simulink model "sampleModel1714_4"  (R2023a)
settings: Solver=VariableStepAuto  StartTime=0.0  StopTime=10.0  RelTol=1e-3
libraries: hdlsllib x5, simulink x2
settings Model: Creator=user1  LastModifiedBy=user1

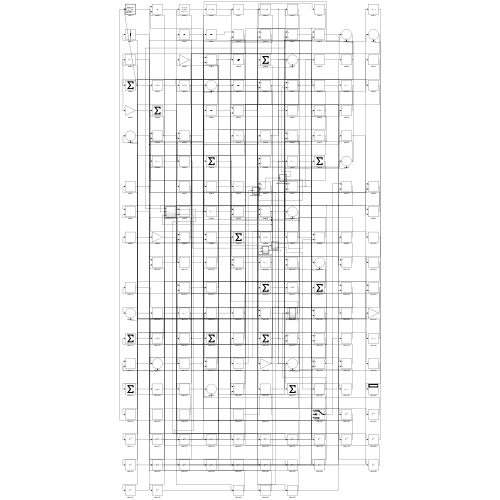
[thumbnail: Simulink's stored preview of the top-level diagram]
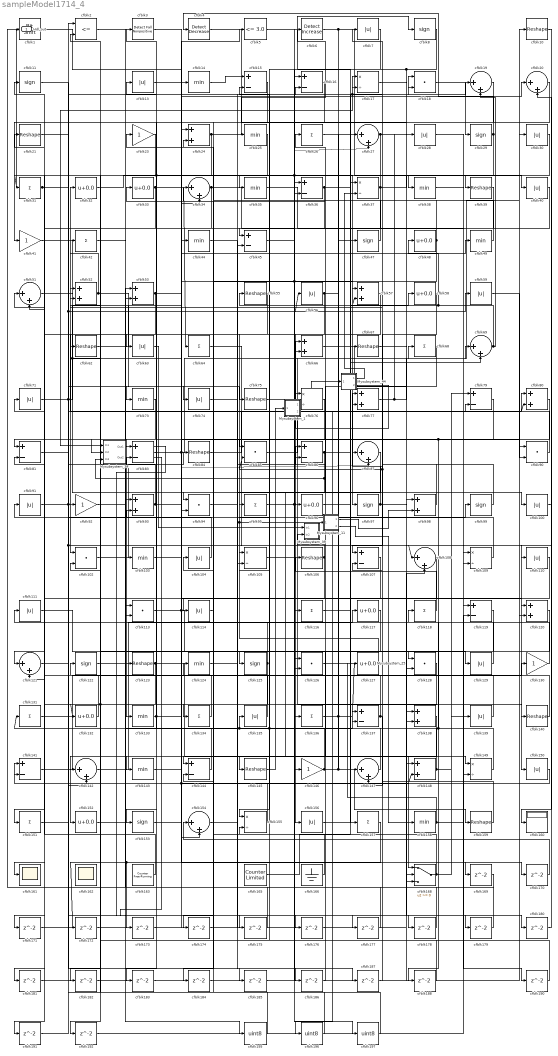
== system sampleModel1714_4 ==
  Mysubsystem_1 : Subsystem  TreatAsAtomicUnit=on  RTWFcnName=Mysubsystem_1
      settings: RTWFcnNameOpts=User specified  RTWFileNameOpts=Use function name
  Mysubsystem_11 : Subsystem  TreatAsAtomicUnit=on  RTWFcnName=Mysubsystem_11
      settings: RTWFcnNameOpts=User specified  RTWFileNameOpts=Use function name
  Mysubsystem_25 : Subsystem  TreatAsAtomicUnit=on  RTWFcnName=Mysubsystem_25
      settings: RTWFcnNameOpts=User specified  RTWFileNameOpts=Use function name
  Mysubsystem_34 : Subsystem  TreatAsAtomicUnit=on  RTWFcnName=Mysubsystem_34
      settings: RTWFcnNameOpts=User specified  RTWFileNameOpts=Use function name
  Mysubsystem_39 : Subsystem  TreatAsAtomicUnit=on  RTWFcnName=Mysubsystem_39
      settings: RTWFcnNameOpts=User specified  RTWFileNameOpts=Use function name
  Mysubsystem_44 : Subsystem  TreatAsAtomicUnit=on  RTWFcnName=Mysubsystem_44
      settings: RTWFcnNameOpts=User specified  RTWFileNameOpts=Use function name
  cfblk1 : hdlsllib/Logic and Bit Operations/Bit Shift  mode=Shift Left Logical  N=0
  cfblk{10,21,39,55,62,67,75,84,106,123,140,145,159} (13 alike) : Reshape
  cfblk{7,13,28,30,40,56,59,63,71,74,91,100,104,110..111,114,129,135,139,150,156} (21 alike) : Abs  OutDataTypeStr=uint8  SaturateOnIntegerOverflow=off
  cfblk{18,85,90,94,102,113,126,128} (8 alike) : DotProduct  OutDataTypeStr=uint8
  cfblk{14,25,35,38,44,49,73,103,124,133,143,158} (12 alike) : MinMax  OutDataTypeStr=uint8
  cfblk{17,37,76,105,109,149,155} (7 alike) : Product  Inputs=*/  OutDataTypeStr=uint8  RndMeth=Zero  SaturateOnIntegerOverflow=on
  cfblk{15..16,36,45,79,81,83,86,107,119,137,141,144} (13 alike) : Sum  Inputs=+-  OutDataTypeStr=uint8
  cfblk{19..20,27,34,51,69,87,108,121,142,147,154} (12 alike) : Sum  Inputs=|++  OutDataTypeStr=uint8
  cfblk{8,11,29,47,97,99,122,125,153} (9 alike) : Signum
  cfblk{26,31,42,64,68,95,116,118,131,134,136,151,157} (13 alike) : Sum  Inputs=+  OutDataTypeStr=uint8
  cfblk{32..33,48,58,96,117,127,132,152} (9 alike) : Bias  Bias=0.0  SaturateOnIntegerOverflow=off
  cfblk{24,52..53,57,66,77,80,93,98,120,138,148} (12 alike) : Sum  OutDataTypeStr=uint8
  cfblk{23,41,92,130,146} (5 alike) : Gain  OutDataTypeStr=uint8
  cfblk160 : Display
  cfblk161 : Scope
  cfblk162 : Scope
      settings: Floating=on
  cfblk163 : hdlsllib/Sources/Counter Free-Running  NumBits=16  tsamp=-1
  cfblk165 : hdlsllib/Sources/Counter Limited  uplimit=7  tsamp=-1
  cfblk166 : Ground
  cfblk168 : Switch  OutDataTypeStr=uint8  SaturateOnIntegerOverflow=off  InputSameDT=off
  cfblk{169..188,190..192} (23 alike) : Delay  SampleTime=1
  cfblk195 : DataTypeConversion  OutDataTypeStr=uint8  SaturateOnIntegerOverflow=off  RndMeth=Floor
  cfblk196 : DataTypeConversion  OutDataTypeStr=uint8  SaturateOnIntegerOverflow=off  RndMeth=Floor
  cfblk197 : DataTypeConversion  OutDataTypeStr=uint8  SaturateOnIntegerOverflow=off  RndMeth=Floor
  cfblk2 : RelationalOperator  Operator=<=  OutDataTypeStr=boolean  InputSameDT=off
  cfblk3 : hdlsllib/Logic and Bit Operations/Detect Fall Nonpositive  vinit=0  OutDataTypeStr=uint8
  cfblk4 : simulink/Logic and Bit Operations/Detect Decrease  vinit=0.0  OutDataTypeStr=uint8
      settings: LibrarySourceBlock=|
      | hdlsllib/Logic and Bit
      | Operations/Detect
      | Decrease
  cfblk5 : hdlsllib/Logic and Bit Operations/Compare To Constant  relop=<=  const=3.0  OutDataTypeStr=uint8
  cfblk6 : simulink/Logic and Bit Operations/Detect Increase  vinit=0.0  OutDataTypeStr=uint8
      settings: LibrarySourceBlock=|
      | hdlsllib/Logic and Bit
      | Operations/Detect
      | Increase
  Hdl_out : Outport  OutDataTypeStr=uint8
  wires:
  cfblk86/1 -> Mysubsystem_34/3(In3), cfblk144/1, cfblk18/2
  cfblk6/1 -> cfblk38/1, cfblk147/1
  cfblk53/1 -> cfblk102/1, cfblk90/2
  cfblk109/1 -> cfblk33/1
  cfblk32/1 -> cfblk97/1
  cfblk150/1 -> cfblk141/1
  cfblk33/1 -> cfblk64/1, cfblk51/2
  cfblk31/1 -> cfblk108/1, cfblk176/1, Hdl_out/1
  cfblk48/1 -> cfblk76/2, cfblk174/1, cfblk24/2
  cfblk142/1 -> cfblk117/1
  cfblk151/1 -> cfblk56/1, cfblk17/2, cfblk92/1
  cfblk114/1 -> cfblk34/1
  cfblk165/1 -> cfblk37/1
  cfblk41/1 -> cfblk73/1
  cfblk137/1 -> cfblk122/1, cfblk147/2
  cfblk129/1 -> cfblk71/1
  cfblk84/1 -> cfblk77/1
  cfblk100/1 -> cfblk160/1
  cfblk121/1 -> cfblk99/1
  cfblk123/1 -> cfblk168/1, cfblk191/1
  cfblk163/1 -> cfblk51/1
  cfblk166/1 -> cfblk105/1
  cfblk57/1 -> cfblk156/1
  cfblk96/1 -> cfblk58/1
  cfblk64/1 -> cfblk150/1
  cfblk87/1 -> cfblk105/2
  cfblk136/1 -> cfblk127/1, cfblk47/1
  cfblk25/1 -> cfblk143/1, cfblk161/1
  cfblk158/1 -> Mysubsystem_25/1(In1), cfblk130/1
  cfblk133/1 -> cfblk13/1, cfblk5/1
  cfblk24/1 -> cfblk8/1, cfblk63/1
  cfblk83/1 -> cfblk25/1, cfblk59/1
  cfblk29/1 -> cfblk4/1, cfblk182/1
  cfblk58/1 -> cfblk107/1
  cfblk26/1 -> cfblk39/1
  cfblk90/1 -> cfblk32/1
  cfblk135/1 -> cfblk91/1
  cfblk138/1 -> cfblk152/1
  cfblk75/1 -> cfblk140/1
  cfblk19/1 -> cfblk41/1
  cfblk10/1 -> cfblk110/1
  cfblk140/1 -> cfblk111/1
  cfblk159/1 -> cfblk52/1, cfblk85/2
  cfblk102/1 -> cfblk84/1
  cfblk108/1 -> cfblk125/1
  cfblk73/1 -> cfblk133/1
  cfblk113/1 -> cfblk128/1, cfblk87/2
  cfblk149/1 -> cfblk131/1, cfblk135/1, cfblk118/1
  cfblk59/1 -> cfblk90/1
  cfblk55/1 -> cfblk114/1
  cfblk42/1 -> cfblk103/1
  cfblk93/1 -> cfblk62/1, cfblk169/1
  cfblk141/1 -> cfblk30/1
  cfblk99/1 -> cfblk55/1
  cfblk85/1 -> cfblk10/1
  cfblk18/1 -> cfblk29/1
  cfblk39/1 -> cfblk155/1
  cfblk51/1 -> cfblk94/1
  cfblk111/1 -> cfblk126/1
  cfblk71/1 -> cfblk14/1, cfblk44/1, cfblk79/2
  cfblk118/1 -> cfblk106/1
  cfblk168/1 -> cfblk124/1, cfblk79/1
  cfblk21/1 -> cfblk75/1
  cfblk74/1 -> cfblk68/1
  cfblk4/1 -> cfblk98/1
  cfblk126/1 -> cfblk80/1
  cfblk52/1 -> cfblk74/1, cfblk42/1
  cfblk23/1 -> cfblk53/2
  cfblk56/1 -> cfblk81/1, cfblk27/1
  cfblk5/1 -> cfblk157/1
  cfblk148/1 -> cfblk95/1, cfblk121/2, cfblk139/1
  cfblk38/1 -> cfblk119/1
  cfblk45/1 -> cfblk6/1
  cfblk127/1 -> cfblk107/2
  cfblk77/1 -> cfblk69/1, cfblk28/1
  cfblk97/1 -> cfblk77/2, cfblk109/2
  cfblk105/1 -> cfblk19/1, cfblk80/2
  cfblk153/1 -> cfblk49/1, cfblk148/2
  cfblk154/1 -> cfblk16/2
  cfblk124/1 -> cfblk86/1
  cfblk30/1 -> cfblk31/1, cfblk36/2
  cfblk69/1 -> cfblk48/1, cfblk57/2, cfblk19/2
  cfblk139/1 -> cfblk87/1
  cfblk62/1 -> cfblk20/1
  cfblk103/1 -> cfblk120/1
  cfblk47/1 -> cfblk23/1
  cfblk146/1 -> cfblk67/1, cfblk159/1, cfblk93/2
  cfblk144/1 -> cfblk52/2
  cfblk134/1 -> cfblk81/2
  cfblk27/1 -> cfblk180/1, cfblk181/1
  cfblk132/1 -> cfblk21/1
  cfblk17/1 -> cfblk148/1
  cfblk36/1 -> cfblk85/1, cfblk129/1
  cfblk143/1 -> cfblk76/1
  cfblk98/1 -> Mysubsystem_34/1(In1), cfblk17/1
  cfblk125/1 -> cfblk3/1, cfblk183/1
  cfblk1/1 -> cfblk154/2
  cfblk131/1 -> cfblk116/1
  cfblk104/1 -> cfblk11/1
  cfblk15/1 -> cfblk134/1
  cfblk147/1 -> cfblk26/1
  cfblk40/1 -> cfblk83/1
  cfblk156/1 -> cfblk18/1
  cfblk67/1 -> cfblk149/1
  cfblk20/1 -> cfblk123/1
  cfblk95/1 -> cfblk27/2, cfblk197/1
  cfblk3/1 -> cfblk57/1
  cfblk106/1 -> Mysubsystem_39/2(In2), cfblk192/1
  cfblk7/1 -> cfblk45/1
  cfblk155/1 -> cfblk141/2
  cfblk68/1 -> cfblk96/1
  cfblk79/1 -> cfblk151/1, cfblk188/1
  cfblk107/1 -> cfblk121/1
  cfblk80/1 -> cfblk94/2
  cfblk116/1 -> cfblk69/2
  cfblk14/1 -> cfblk15/1
  cfblk49/1 -> cfblk7/1
  cfblk16/1 -> cfblk153/1
  cfblk37/1 -> cfblk40/1, cfblk35/1, cfblk145/1
  cfblk130/1 -> cfblk15/2
  cfblk120/1 -> cfblk136/1
  cfblk13/1 -> cfblk100/1
  cfblk152/1 -> cfblk137/1
  cfblk66/1 -> cfblk138/2
  cfblk119/1 -> cfblk142/1, cfblk132/1
  cfblk157/1 -> cfblk172/1, cfblk173/1
  cfblk35/1 -> cfblk109/1
  cfblk8/1 -> cfblk128/2, cfblk66/2
  cfblk91/1 -> cfblk83/2
  cfblk117/1 -> cfblk146/1
  cfblk34/1 -> cfblk126/2, cfblk113/2
  cfblk169/1 -> cfblk1/1
  cfblk94/1 -> cfblk170/1
  cfblk170/1 -> cfblk154/1
  cfblk128/1 -> cfblk171/1
  cfblk171/1 -> cfblk34/2
  cfblk172/1 -> cfblk45/2
  cfblk173/1 -> cfblk168/2
  cfblk174/1 -> cfblk144/2
  cfblk122/1 -> cfblk175/1
  cfblk175/1 -> cfblk24/1
  cfblk176/1 -> cfblk138/1
  cfblk177/1 -> cfblk93/1
  cfblk178/1 -> cfblk16/1
  cfblk11/1 -> cfblk179/1
  cfblk179/1 -> cfblk53/1
  cfblk180/1 -> cfblk20/2
  cfblk181/1 -> cfblk108/2
  cfblk182/1 -> cfblk119/2
  cfblk183/1 -> cfblk168/3
  cfblk110/1 -> cfblk184/1
  cfblk184/1 -> cfblk120/2
  cfblk81/1 -> cfblk185/1
  cfblk185/1 -> cfblk36/1
  cfblk44/1 -> cfblk186/1
  cfblk186/1 -> cfblk86/2
  cfblk92/1 -> cfblk187/1
  cfblk187/1 -> cfblk137/2
  cfblk188/1 -> cfblk155/2
  cfblk28/1 -> cfblk190/1
  cfblk190/1 -> cfblk102/2
  cfblk191/1 -> cfblk142/2
  cfblk192/1 -> cfblk149/2
  cfblk2/1 -> cfblk195/1
  cfblk195/1 -> cfblk104/1
  cfblk196/1 -> cfblk2/1
  cfblk197/1 -> cfblk2/2
  cfblk145/1 -> Mysubsystem_1/1(In1)
  Mysubsystem_1/2(Out2) -> cfblk196/1
  Mysubsystem_11/1(Out1) -> cfblk98/2
  Mysubsystem_11/2(Out2) -> cfblk158/1
  Mysubsystem_25/1(Out1) -> cfblk113/1, Mysubsystem_11/1(In1)
  cfblk76/1 -> Mysubsystem_34/2(In2)
  Mysubsystem_34/1(Out1) -> cfblk177/1
  Mysubsystem_34/2(Out2) -> cfblk178/1
  cfblk63/1 -> Mysubsystem_39/1(In1)
  Mysubsystem_1/1(Out1) -> Mysubsystem_44/1(In1)
  Mysubsystem_44/1(Out1) -> cfblk37/2
  Mysubsystem_44/2(Out2) -> cfblk66/1

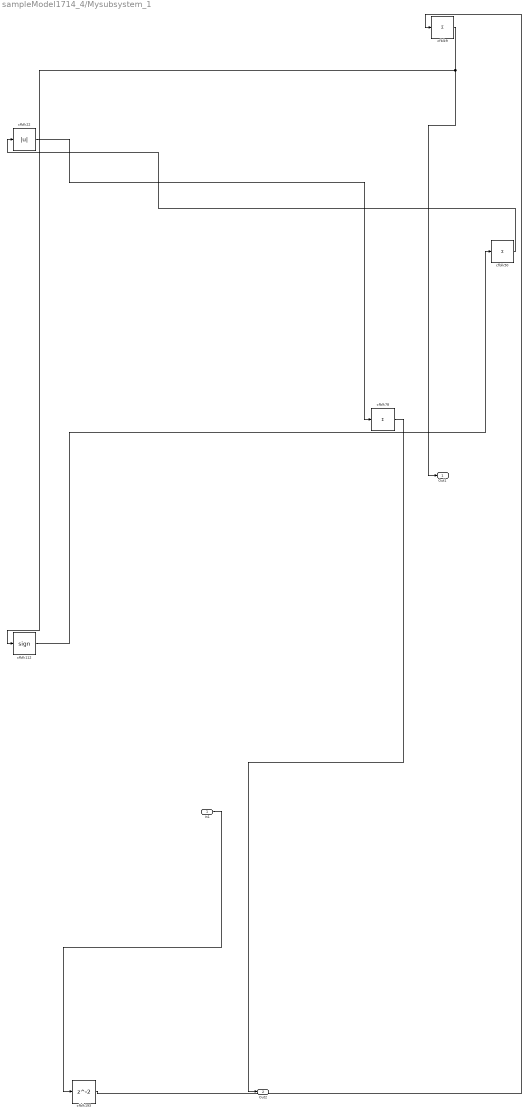
== system sampleModel1714_4/Mysubsystem_1 ==
  In1 : Inport
  cfblk112 : Signum
  cfblk193 : Delay  SampleTime=1
  cfblk22 : Abs  SaturateOnIntegerOverflow=off
  cfblk50 : Sum  Inputs=+
  cfblk78 : Sum  Inputs=+
  cfblk9 : Sum  Inputs=+
  Out1 : Outport
  Out2 : Outport  Port=2
  wires:
  cfblk193/1 -> cfblk9/1
  cfblk9/1 -> Out1/1, cfblk112/1
  cfblk50/1 -> cfblk22/1
  In1/1 -> cfblk193/1
  cfblk22/1 -> cfblk78/1
  cfblk78/1 -> Out2/1
  cfblk112/1 -> cfblk50/1

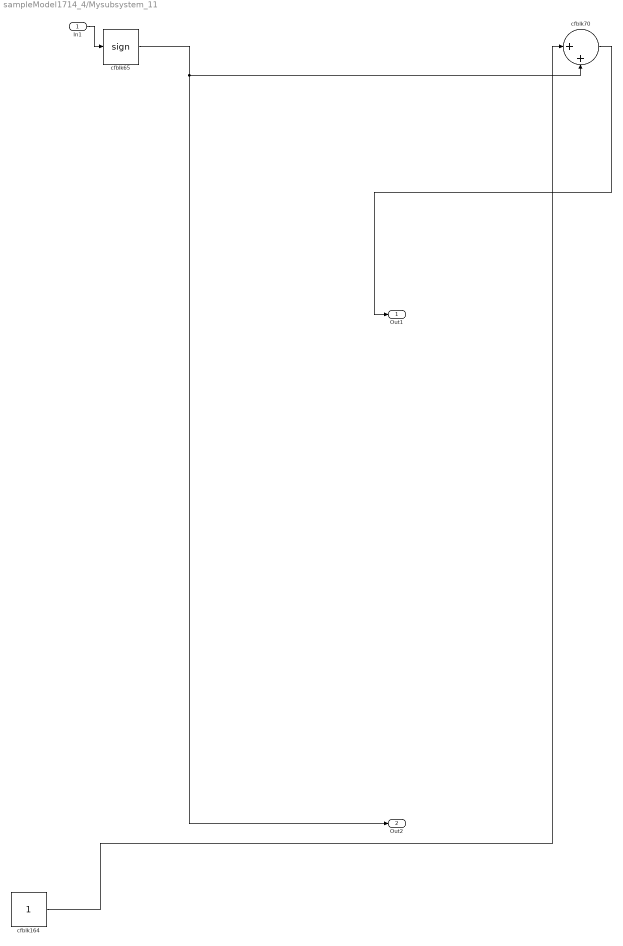
== system sampleModel1714_4/Mysubsystem_11 ==
  In1 : Inport
  cfblk164 : Constant  SampleTime=-1
  cfblk65 : Signum
  cfblk70 : Sum  Inputs=|++
  Out1 : Outport
  Out2 : Outport  Port=2
  wires:
  In1/1 -> cfblk65/1
  cfblk65/1 -> Out2/1, cfblk70/2
  cfblk164/1 -> cfblk70/1
  cfblk70/1 -> Out1/1

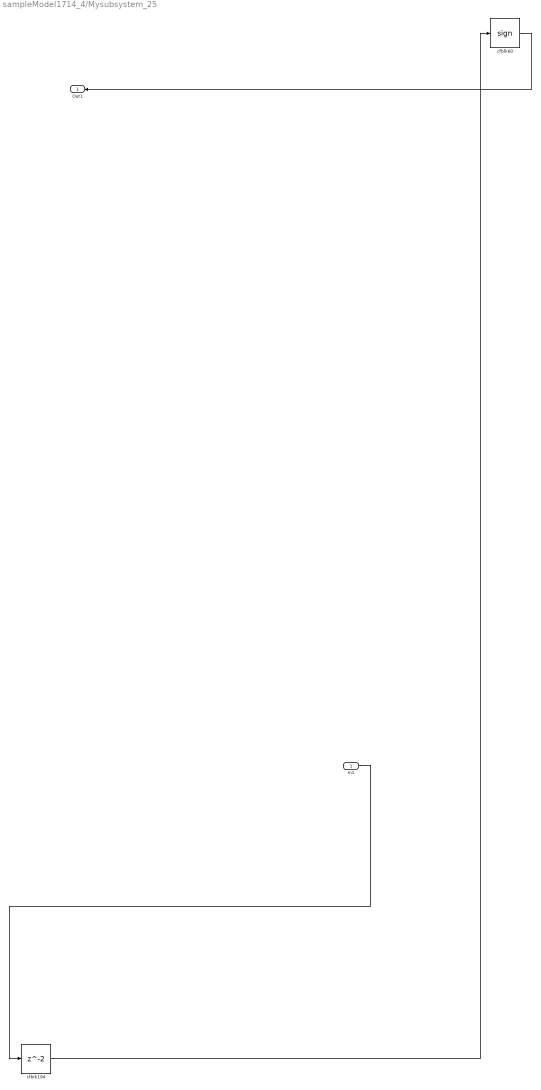
== system sampleModel1714_4/Mysubsystem_25 ==
  In1 : Inport
  cfblk194 : Delay  SampleTime=1
  cfblk60 : Signum
  Out1 : Outport
  wires:
  cfblk194/1 -> cfblk60/1
  cfblk60/1 -> Out1/1
  In1/1 -> cfblk194/1

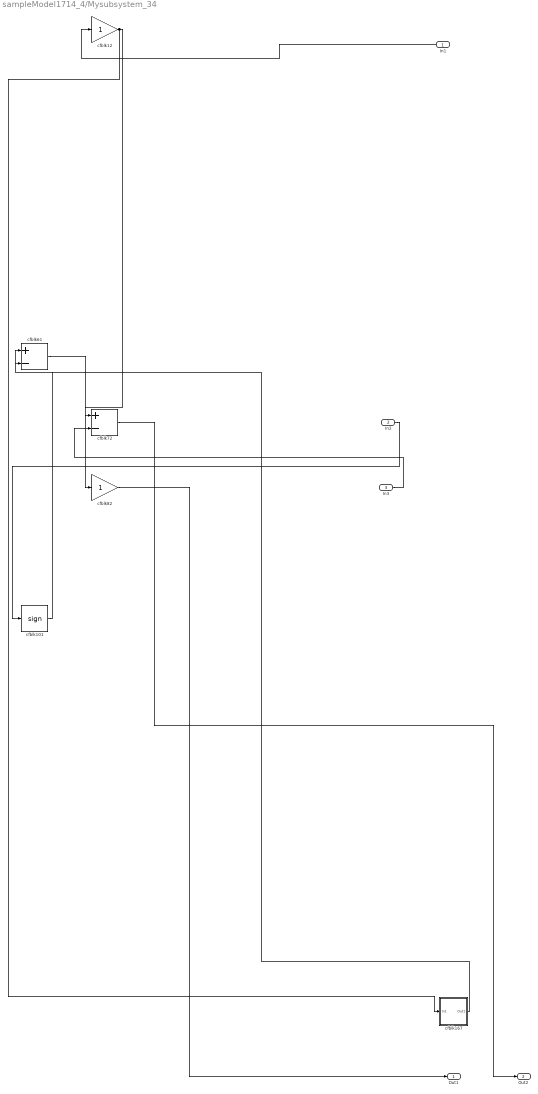
== system sampleModel1714_4/Mysubsystem_34 ==
  In1 : Inport
  In2 : Inport  Port=2
  In3 : Inport  Port=3
  cfblk101 : Signum
  cfblk12 : Gain
  cfblk167 : Subsystem
      settings: LibrarySourceBlock=|
      | hdlsllib/Ports &
      | Subsystems/Subsystem
  cfblk61 : Sum  Inputs=+-
  cfblk72 : Sum  Inputs=+-
  cfblk82 : Gain
  Out1 : Outport
  Out2 : Outport  Port=2
  wires:
  cfblk82/1 -> Out1/1
  cfblk101/1 -> cfblk61/2
  In1/1 -> cfblk12/1
  In2/1 -> cfblk101/1
  cfblk12/1 -> cfblk167/1(In1), cfblk72/1
  cfblk167/1(Out1) -> cfblk61/1
  cfblk61/1 -> cfblk82/1
  In3/1 -> cfblk72/2
  cfblk72/1 -> Out2/1

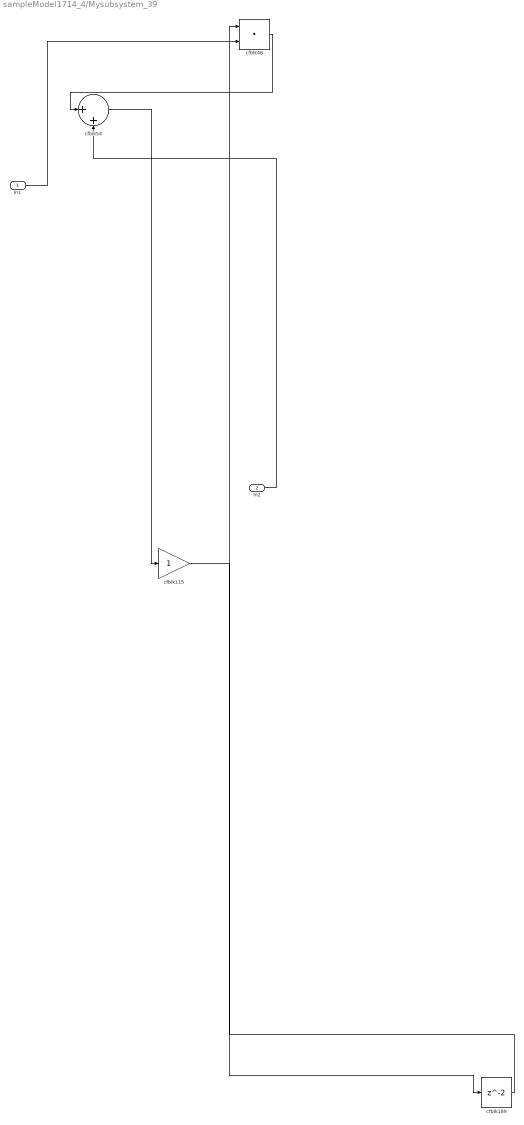
== system sampleModel1714_4/Mysubsystem_39 ==
  In1 : Inport
  In2 : Inport  Port=2
  cfblk115 : Gain
  cfblk189 : Delay  SampleTime=1
  cfblk46 : DotProduct  OutDataTypeStr=Inherit: Inherit via internal rule
  cfblk54 : Sum  Inputs=|++
  wires:
  In1/1 -> cfblk46/2
  cfblk46/1 -> cfblk54/1
  cfblk54/1 -> cfblk115/1
  cfblk189/1 -> cfblk46/1
  cfblk115/1 -> cfblk189/1
  In2/1 -> cfblk54/2

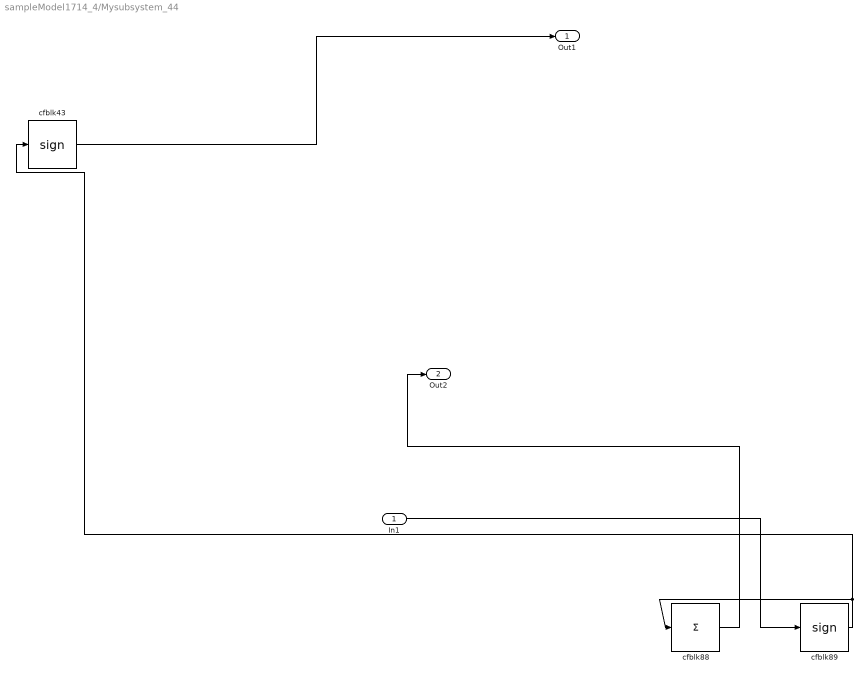
== system sampleModel1714_4/Mysubsystem_44 ==
  In1 : Inport
  cfblk43 : Signum
  cfblk88 : Sum  Inputs=+
  cfblk89 : Signum
  Out1 : Outport
  Out2 : Outport  Port=2
  wires:
  cfblk89/1 -> cfblk88/1, cfblk43/1
  cfblk43/1 -> Out1/1
  cfblk88/1 -> Out2/1
  In1/1 -> cfblk89/1

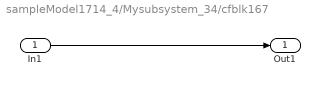
== system sampleModel1714_4/Mysubsystem_34/cfblk167 ==
  In1 : Inport
  Out1 : Outport
  wires:
  In1/1 -> Out1/1
